simulink model "Inverted_pendulum2"  (R2019b)
settings: Solver=VariableStepAuto  StartTime=0.0  StopTime=20  RelTol=1e-3
settings Model: Creator=gongs  LastModifiedBy=gongs
settings DataIOCC: ReturnWorkspaceOutputs=off
settings DebuggingCC: SFMachineParentedDataDiag=error

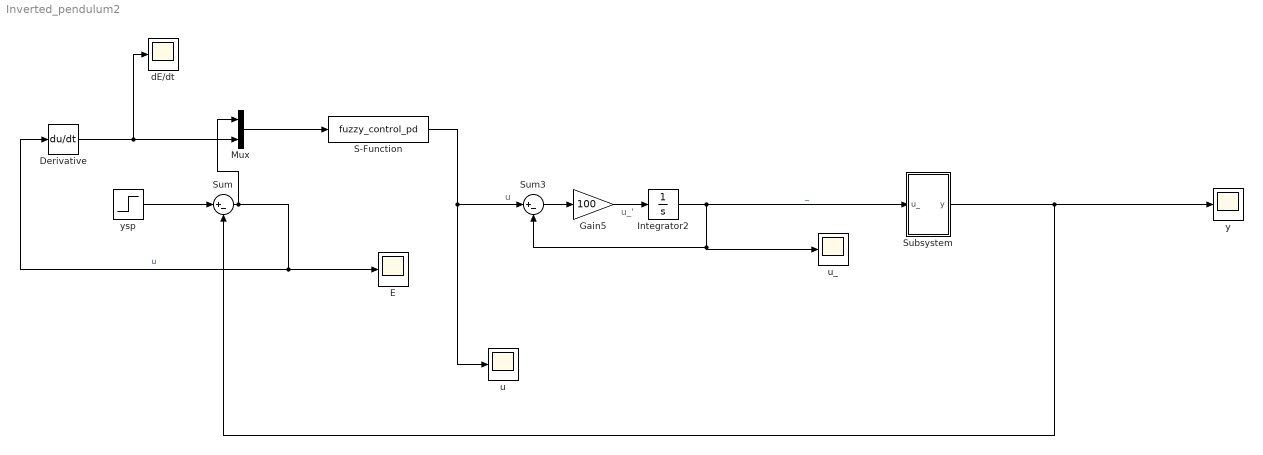
== system Inverted_pendulum2 ==
  note: u
  note: u_'
  Derivative : Derivative
  E : Scope
  Gain5 : Gain  Gain=100
  Integrator2 : Integrator
  Mux : Mux  Inputs=2
  S-Function : S-Function  FunctionName=fuzzy_control_pd  SFunctionDeploymentMode=off  EnableBusSupport=off
  Subsystem : Subsystem
  Sum : Sum  Inputs=|+-
  Sum3 : Sum  Inputs=|+-
  dE/dt : Scope
  u : Scope
  u_ : Scope
  y : Scope
  ysp : Step  Time=0  After=0  SampleTime=0
  wires:
  Sum3/1 -> Gain5/1
  Gain5/1 -> Integrator2/1
  Integrator2/1 -> Subsystem/1(u_), Sum3/2, u_/1  "_"
  Subsystem/1(y) -> y/1, Sum/2
  ysp/1 -> Sum/1
  Sum/1 -> Mux/1, E/1, Derivative/1  "u"
  S-Function/1 -> Sum3/1, u/1
  Mux/1 -> S-Function/1
  Derivative/1 -> dE/dt/1, Mux/2

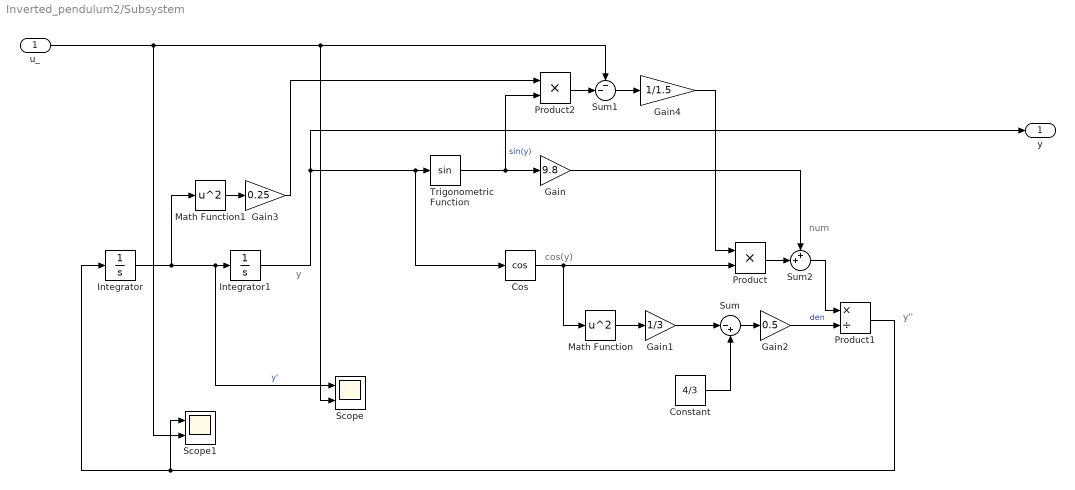
== system Inverted_pendulum2/Subsystem ==
  note: y
  note: y''
  note: num
  note: cos(y)
  u_ : Inport
  Constant : Constant  Value=4/3
  Cos : Trigonometry  Operator=cos
  Gain : Gain  Gain=9.8
  Gain1 : Gain  Gain=1/3
  Gain2 : Gain  Gain=0.5
  Gain3 : Gain  Gain=0.25
  Gain4 : Gain  Gain=1/1.5
  Integrator : Integrator
  Integrator1 : Integrator  InitialCondition=0.1
  Math Function : Math  Operator=square  SignedPower=off  SaturateOnIntegerOverflow=on
  Math Function1 : Math  Operator=square  SignedPower=off  SaturateOnIntegerOverflow=on
  Product : Product
  Product1 : Product  Inputs=*/
  Product2 : Product
  Scope : Scope  NumInputPorts=2
  Scope1 : Scope  NumInputPorts=2
  Sum : Sum  Inputs=|-+
  Sum1 : Sum  Inputs=--|
  Sum2 : Sum  Inputs=++|
  Trigonometric Function : Trigonometry
  y : Outport
  wires:
  Sum/1 -> Gain2/1
  Gain4/1 -> Product/1
  u_/1 -> Scope/2, Sum1/1, Scope1/2
  Cos/1 -> Math Function/1, Product/2
  Product1/1 -> Scope1/1, Integrator/1
  Integrator1/1 -> y/1, Cos/1, Trigonometric Function/1
  Product/1 -> Sum2/2
  Gain2/1 -> Product1/2  "den"
  Math Function1/1 -> Gain3/1
  Sum1/1 -> Gain4/1
  Math Function/1 -> Gain1/1
  Trigonometric Function/1 -> Product2/2, Gain/1  "sin(y)"
  Integrator/1 -> Math Function1/1, Scope/1, Integrator1/1  "y'"
  Product2/1 -> Sum1/2
  Gain3/1 -> Product2/1
  Gain/1 -> Sum2/1
  Constant/1 -> Sum/2
  Gain1/1 -> Sum/1
  Sum2/1 -> Product1/1
